simulink model "S1"  (R2014b)
settings: Solver=ode45  SolverMode=SingleTasking  StartTime=0.0  StopTime=100  MaxStep=5e-3  RelTol=1e-5  AbsTol=1e-5
values from neighbouring files (symbols this model uses):
  Domega = D_fw*Tb/w_b    (= 22.8676282526)    [m1.m]
  fixedFrequency = 0    [m1.m]
  genset = generators(1)    [m1.m]
  H = 5.6    [articlerun.m]    (also in m1.m = 0.5*J_rotor*wbasem*wbasem/Sbase)
  Ki = [-1/Xls 0       0       0       0       0       1/Xls   0 ... (first row only)    [articlerun.m]    (also in m1.m)
  Kmqmd = [ Xaq/Xls 0     0   Xaq/Xlkq2   0       0 ... (first row only)    [articlerun.m]    (also in m1.m = [ Xaq/Xls 0     0   Xaq/Xlkq2 0       0)
  Kpsi = [-rs/Xls 0     0       0       0       0       rs/Xls  0 ... (first row only)    [articlerun.m]    (also in m1.m = wb*Kpsi)
  Kv = [  1       0       0       0       0       0 ... (first row only)    [articlerun.m]    (also in m1.m = wb*Kv)
  Kwpsi = [0 -1   0   0   0   0 ... (first row only)    [articlerun.m]    (also in m1.m = zeros(6))
  psiInit = Psi.signals.values(end,1:7)    [articlerun.m]    (also in init.mat = [-391.464820784 14501.79303 -1.35791716672e-12 -350.14204148; m1.m = psiInit([1 2 3 5 6 7]))
  S_b = 325e6    (= 325000000)    [articlerun.m]    (also in m1.m)
  Sbase = S_b    (= 325000000)    [m1.m]
  ShortCircuitOn = 0    [articlerun.m]    (also in m1.m)
  ShortCircuitStart = 0    [articlerun.m]    (also in m1.m)
  ShortCircuitStop = 0    [articlerun.m]    (also in m1.m)
  swbId = 1    [initDrillingRigMSStoolboxMVM.m]
  Tb = S_b/w_b    (= 862089.275081)    [articlerun.m]    (also in m1.m)
  thetaInit = theta(end)*pi/180    [articlerun.m]    (also in init.mat = 0.0269876819053)
  V_b = 26e3    (= 26000)    [articlerun.m]    (also in m1.m = 20000)
  wb = 60*2*pi    (= 376.991118431)    [articlerun.m]    (also in m1.m)
undefined symbols (not defined in the file or in its folder): nr
undefined symbols (not defined in the file): generators
libraries: genset x4, powerlib x1
settings Model: Creator=andrdahl  LastModifiedBy=torsteinibo
settings DataIOCC: LimitDataPoints=off  SignalLoggingSaveFormat=ModelDataLogs  SaveOutput=off  DSMLogging=off  InspectSignalLogs=on  SaveTime=off
settings OptimizationCC: BlockReduction=off  BooleanDataType=off
settings DebuggingCC: SaveWithParameterizedLinksMsg=none  UnderspecifiedInitializationDetection=Classic  MergeDetectMultiDrivingBlocksExec=none  SignalResolutionControl=TryResolveAllWithWarning  SolverPrmCheckMsg=none  MultiTaskDSMMsg=warning  MultiTaskCondExecSysMsg=none  SignalLabelMismatchMsg=warning  StateNameClashWarn=warning  StrictBusMsg=WarnOnBusTreatedAsVector
settings HardwareCC: TargetUnknown=on
settings RTWCC: IncludeERTFirstTime=on

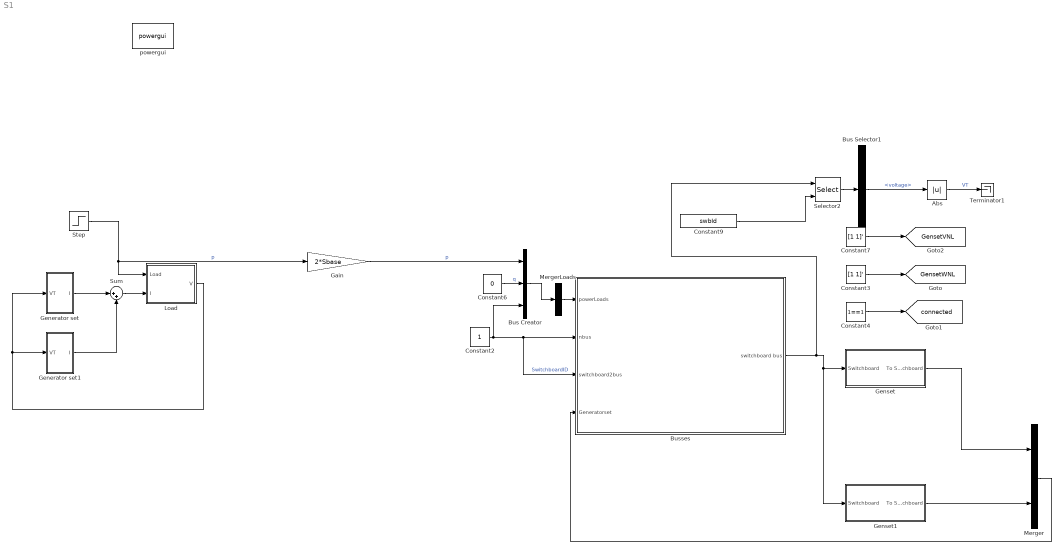
== system S1 ==
  Abs : Abs
  Bus Creator : BusCreator  Inputs='p','q','SwitchboardID'  OutDataTypeStr=Bus: powerLoadsBus  NonVirtualBus=on
  Bus Selector1 : BusSelector  OutputSignals=voltage
  Busses : Subsystem
      mask Display:
      | image(imread('figs/switchboard.jpg'))
      | port_label('input',1,'Power Loads')
      | port_label('input',2,'nbus')
      | port_label('input',3,'switchboard2bus')
      | port_label('input',4,'Generators')
      | port_label('output',1,'switchboard')
  Constant2 : Constant
  Constant3 : Constant  Value=[1 1]'
  Constant4 : Constant  Value=1==1
  Constant6 : Constant  Value=0
  Constant7 : Constant  Value=[1 1]'
  Constant9 : Constant  Value=swbId  OutDataTypeStr=Inherit: Inherit via back propagation
  Gain : Gain  Gain=2*Sbase
  Generator set : Subsystem
  Generator set1 : Subsystem
  Genset : Subsystem  mask{genset=generators(1)}
  Genset1 : Subsystem  mask{genset=generators(2)}
  Load : Subsystem
  Merger : Concatenate  Tag=FromGeneratorsetElectric/Merger
  MergerLoads : Concatenate  Tag=FromLoads/MergerLoads  NumInputs=1
  Selector2 : Selector  IndexOptions=Index vector (port)  Indices=[nr]
  Step : Step  Time=30  Before=.2  After=.7  SampleTime=0
  Sum : Sum  Inputs=|++
  Terminator1 : Terminator
  powergui : powerlib/powergui  Priority=1  SimulationMode=Continuous  SolverType=Tustin  SampleTime=50e-6  frequency=60  SPID=off  DisableSnubberDevices=off  DisableRonSwitches=off  DisableVfSwitches=off  SwTol=0  DisplayEquations=off  Interpol=off  methode=off  Ts=0  frequencyindice=60  Pbase=100e6  ErrMax=1e-4  Iterations=50  UnitsV=kV  UnitsW=MW  FunctionMessages=off  echomessages=off  HookPort=off  EnableUseOfTLC=off  x0status=blocks  RestoreLinks=warning  ResistiveCurrentMeasurement=off  Frange=[0:2:500]  Ylog=off  Xlog=on  ShowGrid=off  save=off  variable=ZData  structure=0  ZoomFFT=off  StartTime=0.0  cycles=1  DisplayStyle=1  fundamental=60  FreqAxis=off  MaxFrequency=1000  frequencyindicesteady=1  RmsSteady=1  display=off
  tag scope: GensetVNL=global, GensetWNL=global, connected=global
  wires:
  Merger/1 -> Busses/4(Generatorset)
  Genset1/1(To Switchboard) -> Merger/2
  Constant2/1 -> Bus Creator/3, Busses/3(switchboard2bus), Busses/2(nbus)  "SwitchboardID"
  Constant3/1 -> [GensetWNL]
  Constant4/1 -> [connected]
  MergerLoads/1 -> Busses/1(powerLoads)
  Bus Creator/1 -> MergerLoads/1
  Step/1 -> Gain/1, Load/1(Load)  "p"
  Constant6/1 -> Bus Creator/2  "q"
  Genset/1(To Switchboard) -> Merger/1
  Constant7/1 -> [GensetVNL]
  Constant9/1 -> Selector2/2
  Busses/1(switchboard bus) -> Selector2/1, Genset1/1(Switchboard), Genset/1(Switchboard)
  Selector2/1 -> Bus Selector1/1
  Bus Selector1/1 -> Abs/1  "<voltage>"
  Abs/1 -> Terminator1/1  "VT"
  Load/1(V) -> Generator set1/1(VT), Generator set/1(VT)
  Generator set/1(I) -> Sum/1
  Gain/1 -> Bus Creator/1  "p"
  Sum/1 -> Load/2(I)
  Generator set1/1(I) -> Sum/2

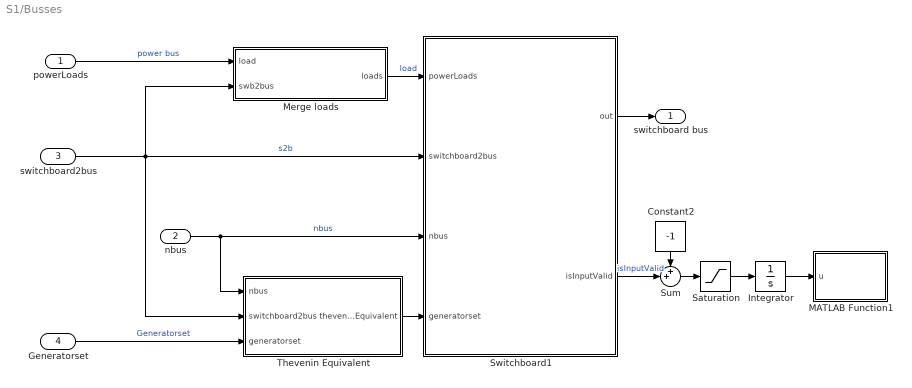
== system S1/Busses ==
  powerLoads : Inport  OutDataTypeStr=Bus: powerLoadsBus
  nbus : Inport  Port=2
  switchboard2bus : Inport  Port=3
  Generatorset : Inport  Port=4
  Constant2 : Constant  Value=-1
  Integrator : Integrator
  MATLAB Function1 : MATLAB Function  TreatAsAtomicUnit=on
  Merge loads : MATLAB Function  TreatAsAtomicUnit=on
  Saturation : Saturate  UpperLimit=0  LowerLimit=-1
  Sum : Sum  Inputs=++|
  Switchboard1 : MATLAB Function  TreatAsAtomicUnit=on
  Thevenin Equivalent : MATLAB Function  TreatAsAtomicUnit=on
  switchboard bus : Outport
  wires:
  Switchboard1/1(out) -> switchboard bus/1
  powerLoads/1 -> Merge loads/1(load)  "power bus"
  switchboard2bus/1 -> Thevenin Equivalent/2(switchboard2bus), Switchboard1/2(switchboard2bus), Merge loads/2(swb2bus)  "s2b"
  Generatorset/1 -> Thevenin Equivalent/3(generatorset)  "Generatorset"
  Integrator/1 -> MATLAB Function1/1(u)
  Constant2/1 -> Sum/1
  Sum/1 -> Saturation/1
  Switchboard1/2(isInputValid) -> Sum/2  "isInputValid"
  nbus/1 -> Thevenin Equivalent/1(nbus), Switchboard1/3(nbus)  "nbus"
  Merge loads/1(loads) -> Switchboard1/1(powerLoads)  "load"
  Thevenin Equivalent/1(theveninEquivalent) -> Switchboard1/4(generatorset)
  Saturation/1 -> Integrator/1

== system S1/Generator set ==
  VT : Inport
  AVR1 : Subsystem  AncestorBlock=PMSlib/Genset/AVR
  Demux4 : Demux  Outputs=3
  Embedded MATLAB Function : MATLAB Function  TreatAsAtomicUnit=on
  Embedded MATLAB Function1 : MATLAB Function  TreatAsAtomicUnit=on
  Embedded MATLAB Function2 : MATLAB Function  TreatAsAtomicUnit=on
  Generator : Subsystem
  Motor : Subsystem
  Product2 : Product  Multiplication=Matrix(*)  RndMeth=Zero
  Product3 : Product  Multiplication=Matrix(*)  RndMeth=Zero
  theta : Integrator  InitialCondition=thetaInit
  I : Outport
  wires:
  AVR1/1(Vf) -> Generator/3(Exfd)
  Product2/1 -> I/1
  Embedded MATLAB Function2/1(Vt) -> AVR1/2("V_T, Bus voltage")
  Embedded MATLAB Function1/1(Kinv) -> Product2/1
  Generator/3(Iqd0s) -> Product2/2
  theta/1 -> Embedded MATLAB Function1/1(theta), Embedded MATLAB Function/1(theta)
  Generator/4(Reactive power) -> AVR1/1("Q, reactive power")
  Generator/1(Electric torque) -> Motor/2(Electric torque)
  Motor/1(we) -> Generator/1(we), theta/1
  Embedded MATLAB Function/1(K) -> Product3/1
  Product3/1 -> Generator/2(Vqd0s)
  VT/1 -> Demux4/1, Product3/2
  Demux4/1 -> Embedded MATLAB Function2/1(Va)
  Demux4/2 -> Embedded MATLAB Function2/2(Vb)
  Demux4/3 -> Embedded MATLAB Function2/3(Vc)
  Generator/2(Active power) -> Motor/1(Active power)

== system S1/Generator set1 ==
  VT : Inport
  AVR1 : Subsystem  AncestorBlock=PMSlib/Genset/AVR
  Demux4 : Demux  Outputs=3
  Embedded MATLAB Function : MATLAB Function  TreatAsAtomicUnit=on
  Embedded MATLAB Function1 : MATLAB Function  TreatAsAtomicUnit=on
  Embedded MATLAB Function2 : MATLAB Function  TreatAsAtomicUnit=on
  Generator : Subsystem
  Motor : Subsystem
  Product2 : Product  Multiplication=Matrix(*)  RndMeth=Zero
  Product3 : Product  Multiplication=Matrix(*)  RndMeth=Zero
  theta : Integrator  InitialCondition=thetaInit
  I : Outport
  wires:
  AVR1/1(Vf) -> Generator/3(Exfd)
  Product2/1 -> I/1
  Embedded MATLAB Function2/1(Vt) -> AVR1/2("V_T, Bus voltage")
  Embedded MATLAB Function1/1(Kinv) -> Product2/1
  Generator/3(Iqd0s) -> Product2/2
  theta/1 -> Embedded MATLAB Function1/1(theta), Embedded MATLAB Function/1(theta)
  Generator/4(Reactive power) -> AVR1/1("Q, reactive power")
  Generator/1(Electric torque) -> Motor/2(Electric torque)
  Motor/1(we) -> Generator/1(we), theta/1
  Embedded MATLAB Function/1(K) -> Product3/1
  Product3/1 -> Generator/2(Vqd0s)
  VT/1 -> Demux4/1, Product3/2
  Demux4/1 -> Embedded MATLAB Function2/1(Va)
  Demux4/2 -> Embedded MATLAB Function2/2(Vb)
  Demux4/3 -> Embedded MATLAB Function2/3(Vc)
  Generator/2(Active power) -> Motor/1(Active power)

== system S1/Genset ==
  Switchboard : Inport
  Genset : Subsystem
  Terminator : Terminator
  To Switchboard : Outport
  wires:
  Genset/1(TheveninBus) -> To Switchboard/1
  Switchboard/1 -> Genset/1(Switchboard)
  Genset/2(GensetToPMS) -> Terminator/1

== system S1/Genset1 ==
  Switchboard : Inport
  Genset : Subsystem
  Terminator : Terminator
  To Switchboard : Outport
  wires:
  Genset/1(TheveninBus) -> To Switchboard/1
  Switchboard/1 -> Genset/1(Switchboard)
  Genset/2(GensetToPMS) -> Terminator/1

== system S1/Load ==
  Load : Inport
  I : Inport  Port=2
  Constant1 : Constant  Value=[0 0 0]
  Gain : Gain  Gain=2*S_b/V_b^2
  Product : Product  Inputs=*/  RndMeth=Zero
  Step1 : Step  Time=ShortCircuitStart  After=-ShortCircuitOn  SampleTime=0
  Step2 : Step  Time=ShortCircuitStop  After=ShortCircuitOn  SampleTime=0
  Sum1 : Sum  Inputs=|++
  Switch : Switch
  V : Outport
  wires:
  I/1 -> Product/1
  Load/1 -> Gain/1
  Product/1 -> Switch/1
  Sum1/1 -> Switch/2
  Step1/1 -> Sum1/1
  Step2/1 -> Sum1/2
  Constant1/1 -> Switch/3
  Switch/1 -> V/1
  Gain/1 -> Product/2

== system S1/Generator set/AVR1 ==
  "Q, reactive power" : Inport
  "V_T, Bus voltage" : Inport  Port=2
  AVR : Subsystem
  Gain1 : Gain  Gain=1/S_b
  Gain2 : Gain  Gain=1/V_b
  Gain3 : Gain  Gain=V_b*sqrt(2/3)
  Vf : Outport
  wires:
  "Q, reactive power"/1 -> Gain1/1
  "V_T, Bus voltage"/1 -> Gain2/1
  AVR/1(Vf) -> Gain3/1  "vf"
  Gain1/1 -> AVR/1("qe, pu")  "q"
  Gain2/1 -> AVR/2("V_T, pu")  "Vt"
  Gain3/1 -> Vf/1

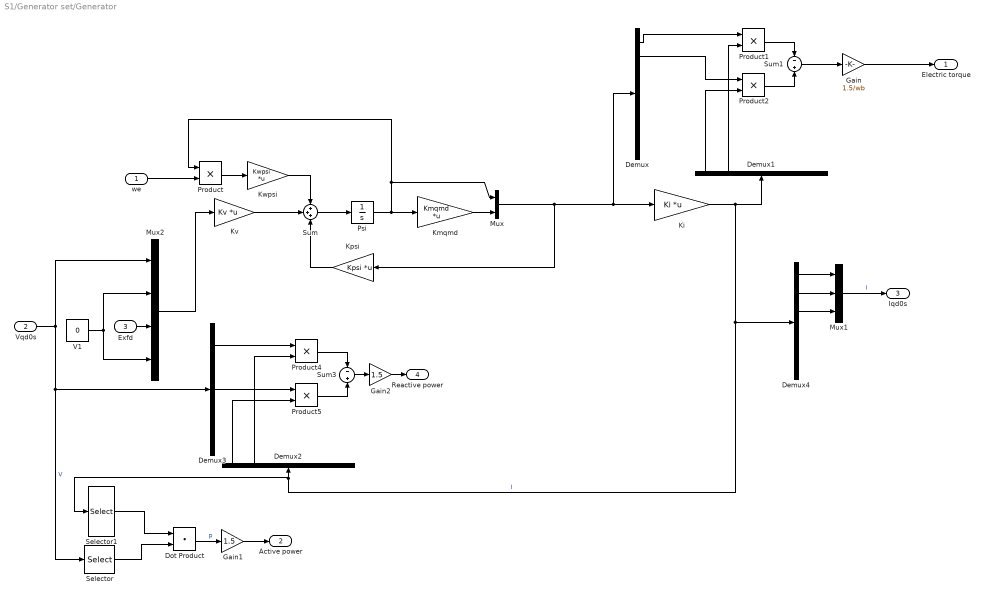
== system S1/Generator set/Generator ==
  we : Inport
  Vqd0s : Inport  Port=2
  Exfd : Inport  Port=3
  Demux : Demux  Outputs=8
  Demux1 : Demux  Outputs=6
  Demux2 : Demux  Outputs=6
  Demux3 : Demux  Outputs=3
  Demux4 : Demux  Outputs=6
  Dot Product : DotProduct  InputSameDT=on  OutDataTypeStr=Inherit: Inherit via internal rule
  Gain : Gain  Gain=1.5/wb
  Gain1 : Gain  Gain=1.5
  Gain2 : Gain  Gain=1.5
  Ki : Gain  Gain=Ki  Multiplication=Matrix(K*u)
  Kmqmd : Gain  Gain=Kmqmd  Multiplication=Matrix(K*u)
  Kpsi : Gain  Gain=Kpsi  Multiplication=Matrix(K*u)
  Kv : Gain  Gain=Kv  Multiplication=Matrix(K*u)
  Kwpsi : Gain  Gain=Kwpsi  Multiplication=Matrix(K*u)
  Mux : Mux  Inputs=2
  Mux1 : Mux  Inputs=3
  Mux2 : Mux
  Product{,1..2,4..5} (5 alike) : Product  RndMeth=Zero
  Psi : Integrator  InitialCondition=psiInit
  Selector : Selector  InputPortWidth=3  Indices=[1 2]
  Selector1 : Selector  InputPortWidth=6  Indices=[1 2]
  Sum : Sum  Inputs=+++
  Sum1 : Sum  Inputs=-+
  Sum3 : Sum  Inputs=-+
  V1 : Constant  Value=0
  Electric torque : Outport
  Active power : Outport  Port=2
  Iqd0s : Outport  Port=3
  Reactive power : Outport  Port=4
  wires:
  Psi/1 -> Kmqmd/1, Mux/1, Product/1
  Sum/1 -> Psi/1
  Product/1 -> Kwpsi/1
  Kwpsi/1 -> Sum/1
  Kv/1 -> Sum/2
  Kpsi/1 -> Sum/3
  Kmqmd/1 -> Mux/2
  Mux/1 -> Kpsi/1, Ki/1, Demux/1
  Ki/1 -> Demux1/1, Selector1/1, Demux2/1, Demux4/1  "I"
  Demux1/2 -> Product1/2
  Demux/1 -> Product1/1
  Demux/2 -> Product2/1
  Demux1/1 -> Product2/2
  Product2/1 -> Sum1/2
  Product1/1 -> Sum1/1
  Mux2/1 -> Kv/1
  Product5/1 -> Sum3/2
  Product4/1 -> Sum3/1
  Demux3/1 -> Product4/1
  Demux2/2 -> Product4/2
  V1/1 -> Mux2/4, Mux2/2
  we/1 -> Product/2
  Vqd0s/1 -> Selector/1, Demux3/1, Mux2/1  "V"
  Exfd/1 -> Mux2/3
  Sum1/1 -> Gain/1
  Sum3/1 -> Gain2/1
  Demux3/2 -> Product5/1
  Demux2/1 -> Product5/2
  Gain/1 -> Electric torque/1
  Demux4/1 -> Mux1/1
  Demux4/2 -> Mux1/2
  Demux4/3 -> Mux1/3
  Mux1/1 -> Iqd0s/1  "I"
  Selector/1 -> Dot Product/2
  Selector1/1 -> Dot Product/1
  Dot Product/1 -> Gain1/1  "p"
  Gain1/1 -> Active power/1
  Gain2/1 -> Reactive power/1

== system S1/Generator set/Motor ==
  Active power : Inport
  Electric torque : Inport  Port=2
  Governor1 : Subsystem
  Inertia : Gain  Gain=wb/(2*H*Tb)  Multiplication=Matrix(K*u)
  Inertia1 : Gain  Gain=1/S_b
  Inertia2 : Gain  Gain=Tb
  Inertia3 : Gain  Gain=1/wb
  Inertia4 : Gain  Gain=Domega  Multiplication=Matrix(K*u)
  Integrator1 : Integrator  InitialCondition=wb
  Sum2 : Sum  Inputs=--+
  we : Outport
  wires:
  Sum2/1 -> Inertia/1
  Inertia/1 -> Integrator1/1
  Integrator1/1 -> Inertia4/1, Inertia3/1, we/1
  Electric torque/1 -> Sum2/2
  Inertia3/1 -> Governor1/1(omega)  "w"
  Inertia2/1 -> Sum2/3
  Active power/1 -> Inertia1/1
  Inertia1/1 -> Governor1/2(P)  "p"
  Governor1/1(u) -> Inertia2/1
  Inertia4/1 -> Sum2/1

== system S1/Generator set1/AVR1 ==
  "Q, reactive power" : Inport
  "V_T, Bus voltage" : Inport  Port=2
  AVR : Subsystem
  Gain1 : Gain  Gain=1/S_b
  Gain2 : Gain  Gain=1/V_b
  Gain3 : Gain  Gain=V_b*sqrt(2/3)
  Vf : Outport
  wires:
  "Q, reactive power"/1 -> Gain1/1
  "V_T, Bus voltage"/1 -> Gain2/1
  AVR/1(Vf) -> Gain3/1  "vf"
  Gain1/1 -> AVR/1("qe, pu")  "q"
  Gain2/1 -> AVR/2("V_T, pu")  "Vt"
  Gain3/1 -> Vf/1

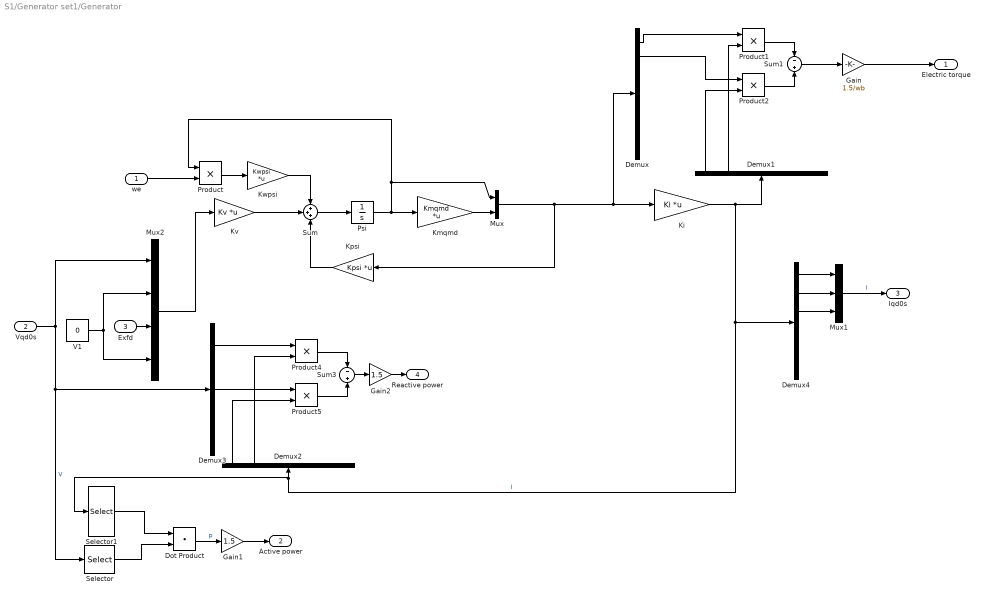
== system S1/Generator set1/Generator ==
  we : Inport
  Vqd0s : Inport  Port=2
  Exfd : Inport  Port=3
  Demux : Demux  Outputs=8
  Demux1 : Demux  Outputs=6
  Demux2 : Demux  Outputs=6
  Demux3 : Demux  Outputs=3
  Demux4 : Demux  Outputs=6
  Dot Product : DotProduct  InputSameDT=on  OutDataTypeStr=Inherit: Inherit via internal rule
  Gain : Gain  Gain=1.5/wb
  Gain1 : Gain  Gain=1.5
  Gain2 : Gain  Gain=1.5
  Ki : Gain  Gain=Ki  Multiplication=Matrix(K*u)
  Kmqmd : Gain  Gain=Kmqmd  Multiplication=Matrix(K*u)
  Kpsi : Gain  Gain=Kpsi  Multiplication=Matrix(K*u)
  Kv : Gain  Gain=Kv  Multiplication=Matrix(K*u)
  Kwpsi : Gain  Gain=Kwpsi  Multiplication=Matrix(K*u)
  Mux : Mux  Inputs=2
  Mux1 : Mux  Inputs=3
  Mux2 : Mux
  Product{,1..2,4..5} (5 alike) : Product  RndMeth=Zero
  Psi : Integrator  InitialCondition=psiInit
  Selector : Selector  InputPortWidth=3  Indices=[1 2]
  Selector1 : Selector  InputPortWidth=6  Indices=[1 2]
  Sum : Sum  Inputs=+++
  Sum1 : Sum  Inputs=-+
  Sum3 : Sum  Inputs=-+
  V1 : Constant  Value=0
  Electric torque : Outport
  Active power : Outport  Port=2
  Iqd0s : Outport  Port=3
  Reactive power : Outport  Port=4
  wires:
  Psi/1 -> Kmqmd/1, Mux/1, Product/1
  Sum/1 -> Psi/1
  Product/1 -> Kwpsi/1
  Kwpsi/1 -> Sum/1
  Kv/1 -> Sum/2
  Kpsi/1 -> Sum/3
  Kmqmd/1 -> Mux/2
  Mux/1 -> Kpsi/1, Ki/1, Demux/1
  Ki/1 -> Demux1/1, Selector1/1, Demux2/1, Demux4/1  "I"
  Demux1/2 -> Product1/2
  Demux/1 -> Product1/1
  Demux/2 -> Product2/1
  Demux1/1 -> Product2/2
  Product2/1 -> Sum1/2
  Product1/1 -> Sum1/1
  Mux2/1 -> Kv/1
  Product5/1 -> Sum3/2
  Product4/1 -> Sum3/1
  Demux3/1 -> Product4/1
  Demux2/2 -> Product4/2
  V1/1 -> Mux2/4, Mux2/2
  we/1 -> Product/2
  Vqd0s/1 -> Selector/1, Demux3/1, Mux2/1  "V"
  Exfd/1 -> Mux2/3
  Sum1/1 -> Gain/1
  Sum3/1 -> Gain2/1
  Demux3/2 -> Product5/1
  Demux2/1 -> Product5/2
  Gain/1 -> Electric torque/1
  Demux4/1 -> Mux1/1
  Demux4/2 -> Mux1/2
  Demux4/3 -> Mux1/3
  Mux1/1 -> Iqd0s/1  "I"
  Selector/1 -> Dot Product/2
  Selector1/1 -> Dot Product/1
  Dot Product/1 -> Gain1/1  "p"
  Gain1/1 -> Active power/1
  Gain2/1 -> Reactive power/1

== system S1/Generator set1/Motor ==
  Active power : Inport
  Electric torque : Inport  Port=2
  Governor1 : Subsystem
  Inertia : Gain  Gain=wb/(2*H*Tb)  Multiplication=Matrix(K*u)
  Inertia1 : Gain  Gain=1/S_b
  Inertia2 : Gain  Gain=Tb
  Inertia3 : Gain  Gain=1/wb
  Inertia4 : Gain  Gain=Domega  Multiplication=Matrix(K*u)
  Integrator1 : Integrator  InitialCondition=wb
  Sum2 : Sum  Inputs=--+
  we : Outport
  wires:
  Sum2/1 -> Inertia/1
  Inertia/1 -> Integrator1/1
  Integrator1/1 -> Inertia4/1, Inertia3/1, we/1
  Electric torque/1 -> Sum2/2
  Inertia3/1 -> Governor1/1(omega)  "w"
  Inertia2/1 -> Sum2/3
  Active power/1 -> Inertia1/1
  Inertia1/1 -> Governor1/2(P)  "p"
  Governor1/1(u) -> Inertia2/1
  Inertia4/1 -> Sum2/1

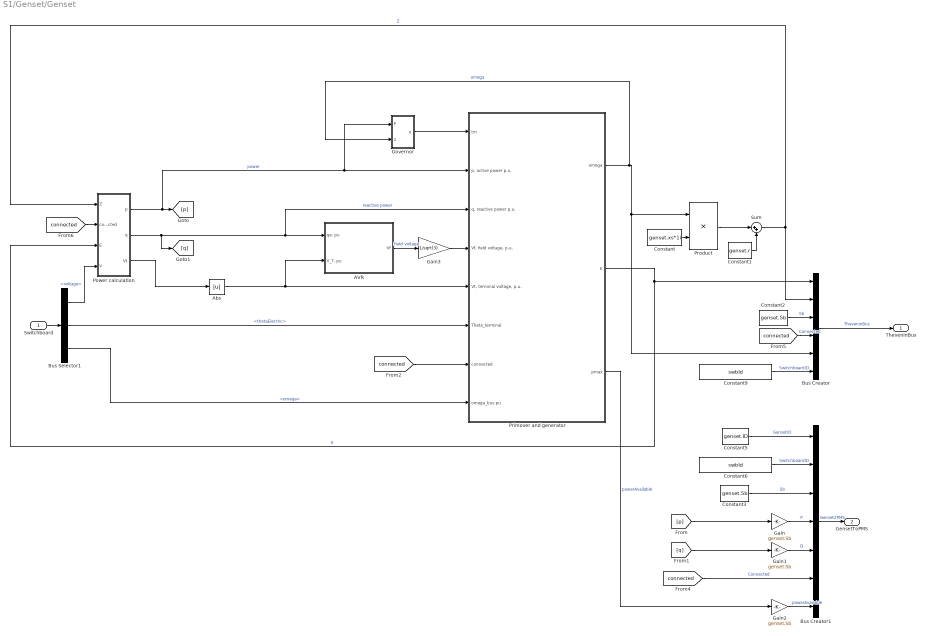
== system S1/Genset/Genset ==
  Switchboard : Inport
  AVR : Subsystem
  Abs : Abs
  Bus Creator : BusCreator  Inputs='E','Z','Sb','Connected','omega','SwitchboardID'  OutDataTypeStr=Bus: TheveninBus  NonVirtualBus=on
  Bus Creator1 : BusCreator  Inputs='GensetID','SwitchboardID','Sb','P','Q','Connected','powerAvailable'  OutDataTypeStr=Bus: Genset2PMS  NonVirtualBus=on
  Bus Selector1 : BusSelector  OutputSignals=voltage,thetaElectric,omega
  Constant : Constant  Value=genset.xs*1i
  Constant1 : Constant  Value=genset.r
  Constant2 : Constant  Value=genset.Sb
  Constant3 : Constant  Value=genset.Sb
  Constant5 : Constant  Value=genset.ID  OutDataTypeStr=Inherit: Inherit via back propagation
  Constant6 : Constant  Value=swbId  OutDataTypeStr=Inherit: Inherit via back propagation
  Constant9 : Constant  Value=swbId  OutDataTypeStr=Inherit: Inherit via back propagation
  Gain : Gain  Gain=genset.Sb
  Gain1 : Gain  Gain=genset.Sb
  Gain2 : Gain  Gain=genset.Sb
  Gain3 : Gain  Gain=1/sqrt(3)
  Governor : Subsystem
  Power calculation : MATLAB Function  TreatAsAtomicUnit=on
  Primover and generator : Subsystem
  Product : Product
  Sum : Sum  Inputs=|++
  TheveninBus : Outport
  GensetToPMS : Outport  Port=2
  wires:
  Bus Creator1/1 -> GensetToPMS/1  "Genset2PMS"
  [p] -> Gain/1
  [q] -> Gain1/1
  Constant2/1 -> Bus Creator/3  "Sb"
  Bus Creator/1 -> TheveninBus/1  "TheveninBus"
  Sum/1 -> Bus Creator/2, Power calculation/1(Z)  "Z"
  Constant1/1 -> Sum/2
  Product/1 -> Sum/1
  Constant/1 -> Product/2
  Abs/1 -> AVR/2("V_T, pu"), Primover and generator/5("Vt, terminal voltage, p.u.")
  Primover and generator/3(pmax) -> Gain2/1  "powerAvailable"
  Power calculation/2(q) -> [q], AVR/1("qe, pu"), Primover and generator/3("q, reactive power p.u.")  "reactive power"
  Power calculation/1(p) -> [p], Governor/1(P), Primover and generator/2("p, active power p.u.")  "power"
  Governor/1(u) -> Primover and generator/1(tm)
  Primover and generator/2(E) -> Power calculation/3(E), Bus Creator/1  "E"
  Primover and generator/1(omega) -> Governor/2(omega), Bus Creator/5, Product/1  "omega"
  AVR/1(Vf) -> Gain3/1  "Field voltage"
  Constant3/1 -> Bus Creator1/3  "Sb"
  Constant5/1 -> Bus Creator1/1  "GensetID"
  Constant6/1 -> Bus Creator1/2  "SwitchboardID"
  Gain/1 -> Bus Creator1/4  "P"
  Gain1/1 -> Bus Creator1/5  "Q"
  Bus Selector1/1 -> Power calculation/4(V)  "<voltage>"
  Gain2/1 -> Bus Creator1/7  "powerAvailable"
  [connected] -> Primover and generator/7(connected)
  [connected] -> Power calculation/2(connected)
  [connected] -> Bus Creator1/6  "Connected"
  [connected] -> Bus Creator/4  "Connected"
  Power calculation/3(Vt) -> Abs/1
  Bus Selector1/3 -> Primover and generator/8(omega_bus pu)  "<omega>"
  Switchboard/1 -> Bus Selector1/1
  Constant9/1 -> Bus Creator/6  "SwitchboardID"
  Bus Selector1/2 -> Primover and generator/6(Theta_terminal)  "<thetaElectric>"
  Gain3/1 -> Primover and generator/4("Vf, field voltage, p.u.")

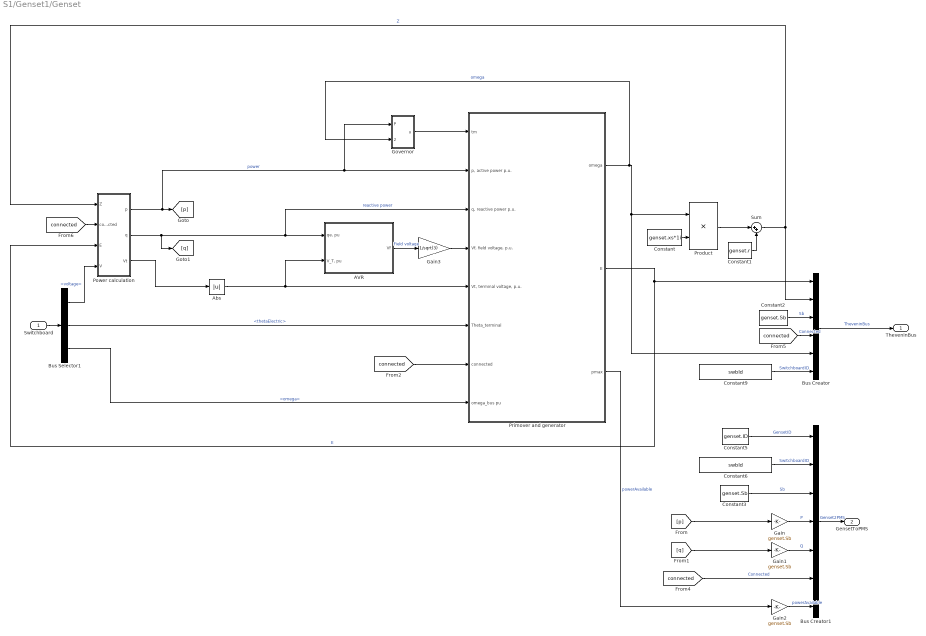
== system S1/Genset1/Genset ==
  Switchboard : Inport
  AVR : Subsystem
  Abs : Abs
  Bus Creator : BusCreator  Inputs='E','Z','Sb','Connected','omega','SwitchboardID'  OutDataTypeStr=Bus: TheveninBus  NonVirtualBus=on
  Bus Creator1 : BusCreator  Inputs='GensetID','SwitchboardID','Sb','P','Q','Connected','powerAvailable'  OutDataTypeStr=Bus: Genset2PMS  NonVirtualBus=on
  Bus Selector1 : BusSelector  OutputSignals=voltage,thetaElectric,omega
  Constant : Constant  Value=genset.xs*1i
  Constant1 : Constant  Value=genset.r
  Constant2 : Constant  Value=genset.Sb
  Constant3 : Constant  Value=genset.Sb
  Constant5 : Constant  Value=genset.ID  OutDataTypeStr=Inherit: Inherit via back propagation
  Constant6 : Constant  Value=swbId  OutDataTypeStr=Inherit: Inherit via back propagation
  Constant9 : Constant  Value=swbId  OutDataTypeStr=Inherit: Inherit via back propagation
  Gain : Gain  Gain=genset.Sb
  Gain1 : Gain  Gain=genset.Sb
  Gain2 : Gain  Gain=genset.Sb
  Gain3 : Gain  Gain=1/sqrt(3)
  Governor : Subsystem
  Power calculation : MATLAB Function  TreatAsAtomicUnit=on
  Primover and generator : Subsystem
  Product : Product
  Sum : Sum  Inputs=|++
  TheveninBus : Outport
  GensetToPMS : Outport  Port=2
  wires:
  Bus Creator1/1 -> GensetToPMS/1  "Genset2PMS"
  [p] -> Gain/1
  [q] -> Gain1/1
  Constant2/1 -> Bus Creator/3  "Sb"
  Bus Creator/1 -> TheveninBus/1  "TheveninBus"
  Sum/1 -> Bus Creator/2, Power calculation/1(Z)  "Z"
  Constant1/1 -> Sum/2
  Product/1 -> Sum/1
  Constant/1 -> Product/2
  Abs/1 -> AVR/2("V_T, pu"), Primover and generator/5("Vt, terminal voltage, p.u.")
  Primover and generator/3(pmax) -> Gain2/1  "powerAvailable"
  Power calculation/2(q) -> [q], AVR/1("qe, pu"), Primover and generator/3("q, reactive power p.u.")  "reactive power"
  Power calculation/1(p) -> [p], Governor/1(P), Primover and generator/2("p, active power p.u.")  "power"
  Governor/1(u) -> Primover and generator/1(tm)
  Primover and generator/2(E) -> Power calculation/3(E), Bus Creator/1  "E"
  Primover and generator/1(omega) -> Governor/2(omega), Bus Creator/5, Product/1  "omega"
  AVR/1(Vf) -> Gain3/1  "Field voltage"
  Constant3/1 -> Bus Creator1/3  "Sb"
  Constant5/1 -> Bus Creator1/1  "GensetID"
  Constant6/1 -> Bus Creator1/2  "SwitchboardID"
  Gain/1 -> Bus Creator1/4  "P"
  Gain1/1 -> Bus Creator1/5  "Q"
  Bus Selector1/1 -> Power calculation/4(V)  "<voltage>"
  Gain2/1 -> Bus Creator1/7  "powerAvailable"
  [connected] -> Primover and generator/7(connected)
  [connected] -> Power calculation/2(connected)
  [connected] -> Bus Creator1/6  "Connected"
  [connected] -> Bus Creator/4  "Connected"
  Power calculation/3(Vt) -> Abs/1
  Bus Selector1/3 -> Primover and generator/8(omega_bus pu)  "<omega>"
  Switchboard/1 -> Bus Selector1/1
  Constant9/1 -> Bus Creator/6  "SwitchboardID"
  Bus Selector1/2 -> Primover and generator/6(Theta_terminal)  "<thetaElectric>"
  Gain3/1 -> Primover and generator/4("Vf, field voltage, p.u.")

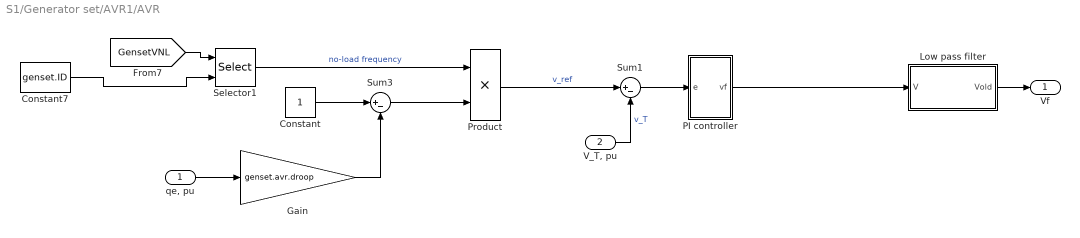
== system S1/Generator set/AVR1/AVR ==
  "qe, pu" : Inport
  "V_T, pu" : Inport  Port=2
  Constant : Constant
  Constant7 : Constant  Value=genset.ID  OutDataTypeStr=Inherit: Inherit via back propagation
  Gain : Gain  Gain=genset.avr.droop
  Low pass filter : Subsystem
  PI controller : Subsystem
  Product : Product  RndMeth=Zero
  Selector1 : Selector  IndexOptions=Index vector (port)  Indices=[nr]
  Sum1 : Sum  Inputs=|+-
  Sum3 : Sum  Inputs=|+-
  Vf : Outport
  wires:
  Low pass filter/1(Vold) -> Vf/1
  Product/1 -> Sum1/1  "v_ref"
  Sum3/1 -> Product/2
  Gain/1 -> Sum3/2
  Constant/1 -> Sum3/1
  "V_T, pu"/1 -> Sum1/2  "v_T"
  "qe, pu"/1 -> Gain/1
  Sum1/1 -> PI controller/1(e)
  Constant7/1 -> Selector1/2
  [GensetVNL] -> Selector1/1
  Selector1/1 -> Product/1  "no-load frequency"
  PI controller/1(vf) -> Low pass filter/1(V)

== system S1/Generator set/Motor/Governor1 ==
  omega : Inport
  P : Inport  Port=2
  Constant : Constant  Value=1/(1-genset.governor.droop*.5)
  Governor : genset/Genset/Governor
  u : Outport
  wires:
  P/1 -> Governor/4
  omega/1 -> Governor/2
  Constant/1 -> Governor/3
  Governor/1 -> u/1, Governor/1

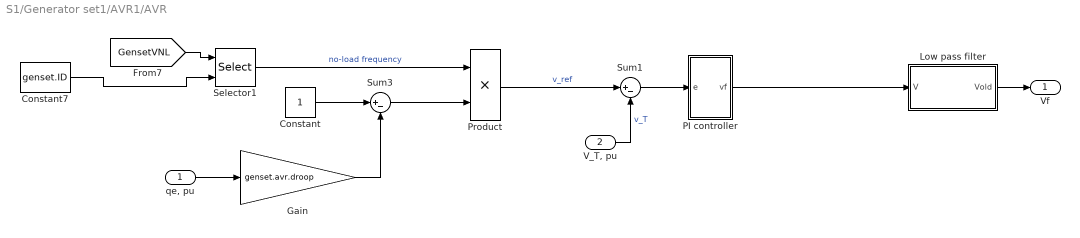
== system S1/Generator set1/AVR1/AVR ==
  "qe, pu" : Inport
  "V_T, pu" : Inport  Port=2
  Constant : Constant
  Constant7 : Constant  Value=genset.ID  OutDataTypeStr=Inherit: Inherit via back propagation
  Gain : Gain  Gain=genset.avr.droop
  Low pass filter : Subsystem
  PI controller : Subsystem
  Product : Product  RndMeth=Zero
  Selector1 : Selector  IndexOptions=Index vector (port)  Indices=[nr]
  Sum1 : Sum  Inputs=|+-
  Sum3 : Sum  Inputs=|+-
  Vf : Outport
  wires:
  Low pass filter/1(Vold) -> Vf/1
  Product/1 -> Sum1/1  "v_ref"
  Sum3/1 -> Product/2
  Gain/1 -> Sum3/2
  Constant/1 -> Sum3/1
  "V_T, pu"/1 -> Sum1/2  "v_T"
  "qe, pu"/1 -> Gain/1
  Sum1/1 -> PI controller/1(e)
  Constant7/1 -> Selector1/2
  [GensetVNL] -> Selector1/1
  Selector1/1 -> Product/1  "no-load frequency"
  PI controller/1(vf) -> Low pass filter/1(V)

== system S1/Generator set1/Motor/Governor1 ==
  omega : Inport
  P : Inport  Port=2
  Constant : Constant  Value=1/(1-genset.governor.droop*.5)
  Governor : genset/Genset/Governor
  u : Outport
  wires:
  P/1 -> Governor/4
  omega/1 -> Governor/2
  Constant/1 -> Governor/3
  Governor/1 -> u/1, Governor/1

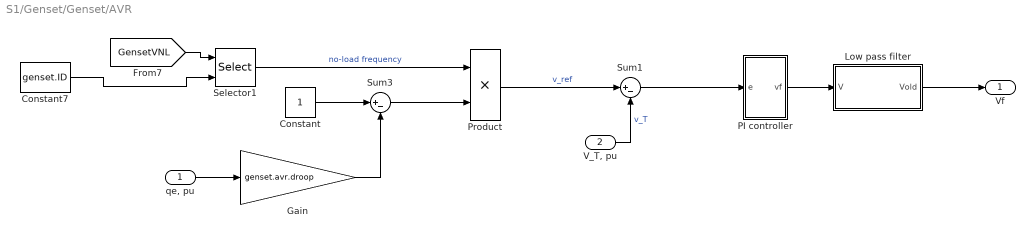
== system S1/Genset/Genset/AVR ==
  "qe, pu" : Inport
  "V_T, pu" : Inport  Port=2
  Constant : Constant
  Constant7 : Constant  Value=genset.ID  OutDataTypeStr=Inherit: Inherit via back propagation
  Gain : Gain  Gain=genset.avr.droop
  Low pass filter : Subsystem
  PI controller : Subsystem
  Product : Product  RndMeth=Zero
  Selector1 : Selector  IndexOptions=Index vector (port)  Indices=[nr]
  Sum1 : Sum  Inputs=|+-
  Sum3 : Sum  Inputs=|+-
  Vf : Outport
  wires:
  Low pass filter/1(Vold) -> Vf/1
  Product/1 -> Sum1/1  "v_ref"
  Sum3/1 -> Product/2
  Gain/1 -> Sum3/2
  Constant/1 -> Sum3/1
  "V_T, pu"/1 -> Sum1/2  "v_T"
  "qe, pu"/1 -> Gain/1
  Sum1/1 -> PI controller/1(e)
  PI controller/1(vf) -> Low pass filter/1(V)
  Constant7/1 -> Selector1/2
  [GensetVNL] -> Selector1/1
  Selector1/1 -> Product/1  "no-load frequency"

== system S1/Genset/Genset/Governor ==
  P : Inport
  omega : Inport  Port=2
  Constant : Constant  Value=1/(1-genset.governor.droop*.5)
  Governor : genset/Genset/Governor
  u : Outport
  wires:
  P/1 -> Governor/4
  omega/1 -> Governor/2
  Constant/1 -> Governor/3
  Governor/1 -> u/1, Governor/1

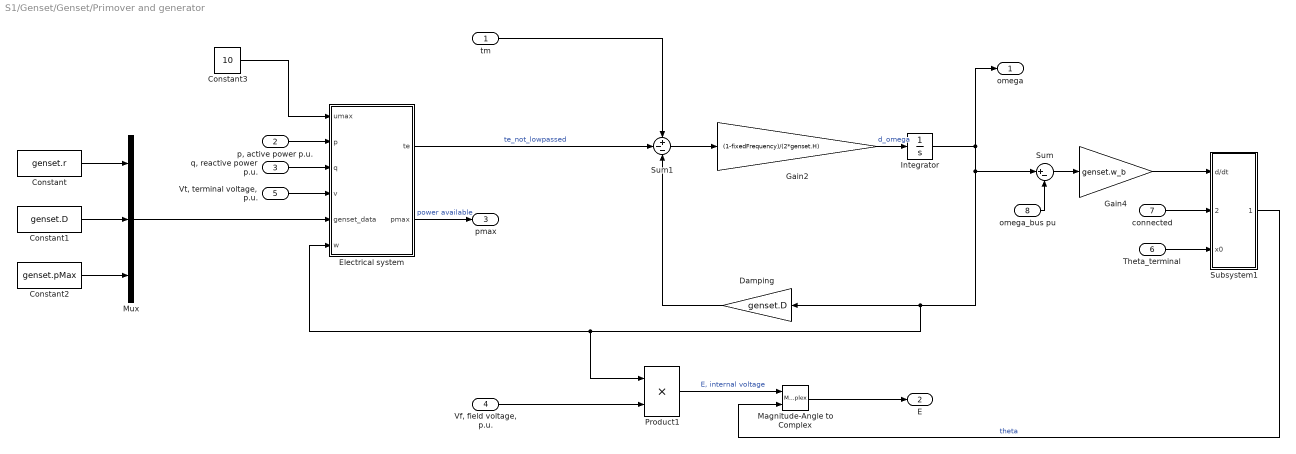
== system S1/Genset/Genset/Primover and generator ==
  tm : Inport
  "p, active power p.u." : Inport  Port=2
  "q, reactive power p.u." : Inport  Port=3
  "Vf, field voltage, p.u." : Inport  Port=4
  "Vt, terminal voltage, p.u." : Inport  Port=5
  Theta_terminal : Inport  Port=6
  connected : Inport  Port=7
  omega_bus pu : Inport  Port=8
  Constant : Constant  Value=genset.r
  Constant1 : Constant  Value=genset.D
  Constant2 : Constant  Value=genset.pMax
  Constant3 : Constant  Value=10
  Damping : Gain  Gain=genset.D
  Electrical system : MATLAB Function  TreatAsAtomicUnit=on
  Gain2 : Gain  Gain=(1-fixedFrequency)/(2*genset.H)
  Gain4 : Gain  Gain=genset.w_b
  Integrator : Integrator  InitialCondition=genset.omega0
  Magnitude-Angle to Complex : MagnitudeAngleToComplex
  Mux : Mux  Inputs=3
  Product1 : Product  Inputs=**  RndMeth=Zero
  Subsystem1 : Subsystem
  Sum : Sum  Inputs=|+-
  Sum1 : Sum  Inputs=+--
  omega : Outport
  E : Outport  Port=2
  pmax : Outport  Port=3
  wires:
  Mux/1 -> Electrical system/5(genset_data)
  Constant2/1 -> Mux/3
  Constant1/1 -> Mux/2
  Constant/1 -> Mux/1
  Magnitude-Angle to Complex/1 -> E/1
  Electrical system/2(pmax) -> pmax/1  "power available"
  Theta_terminal/1 -> Subsystem1/3(x0)
  Integrator/1 -> omega/1, Electrical system/6(w), Product1/1, Damping/1, Sum/1
  connected/1 -> Subsystem1/2(reset)
  Damping/1 -> Sum1/3
  "q, reactive power p.u."/1 -> Electrical system/3(q)
  "Vt, terminal voltage, p.u."/1 -> Electrical system/4(v)
  Electrical system/1(te) -> Sum1/2  "te_not_lowpassed"
  "p, active power p.u."/1 -> Electrical system/2(p)
  "Vf, field voltage, p.u."/1 -> Product1/2
  Gain2/1 -> Integrator/1  "d_omega"
  Sum1/1 -> Gain2/1
  Gain4/1 -> Subsystem1/1(d/dt)
  Subsystem1/1(Out1) -> Magnitude-Angle to Complex/2  "theta"
  Product1/1 -> Magnitude-Angle to Complex/1  "E, internal voltage"
  tm/1 -> Sum1/1
  Sum/1 -> Gain4/1
  omega_bus pu/1 -> Sum/2
  Constant3/1 -> Electrical system/1(umax)

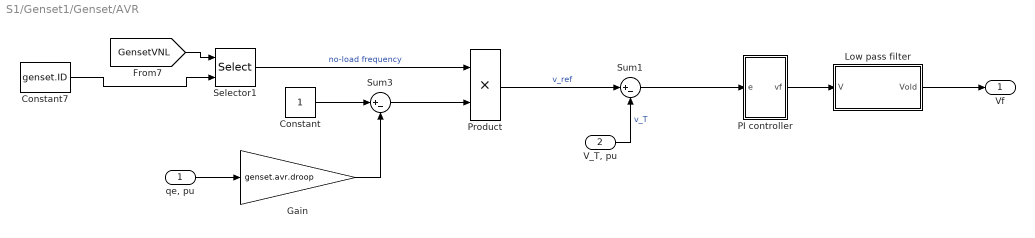
== system S1/Genset1/Genset/AVR ==
  "qe, pu" : Inport
  "V_T, pu" : Inport  Port=2
  Constant : Constant
  Constant7 : Constant  Value=genset.ID  OutDataTypeStr=Inherit: Inherit via back propagation
  Gain : Gain  Gain=genset.avr.droop
  Low pass filter : Subsystem
  PI controller : Subsystem
  Product : Product  RndMeth=Zero
  Selector1 : Selector  IndexOptions=Index vector (port)  Indices=[nr]
  Sum1 : Sum  Inputs=|+-
  Sum3 : Sum  Inputs=|+-
  Vf : Outport
  wires:
  Low pass filter/1(Vold) -> Vf/1
  Product/1 -> Sum1/1  "v_ref"
  Sum3/1 -> Product/2
  Gain/1 -> Sum3/2
  Constant/1 -> Sum3/1
  "V_T, pu"/1 -> Sum1/2  "v_T"
  "qe, pu"/1 -> Gain/1
  Sum1/1 -> PI controller/1(e)
  PI controller/1(vf) -> Low pass filter/1(V)
  Constant7/1 -> Selector1/2
  [GensetVNL] -> Selector1/1
  Selector1/1 -> Product/1  "no-load frequency"

== system S1/Genset1/Genset/Governor ==
  P : Inport
  omega : Inport  Port=2
  Constant : Constant  Value=1/(1-genset.governor.droop*.5)
  Governor : genset/Genset/Governor
  u : Outport
  wires:
  P/1 -> Governor/4
  omega/1 -> Governor/2
  Constant/1 -> Governor/3
  Governor/1 -> u/1, Governor/1

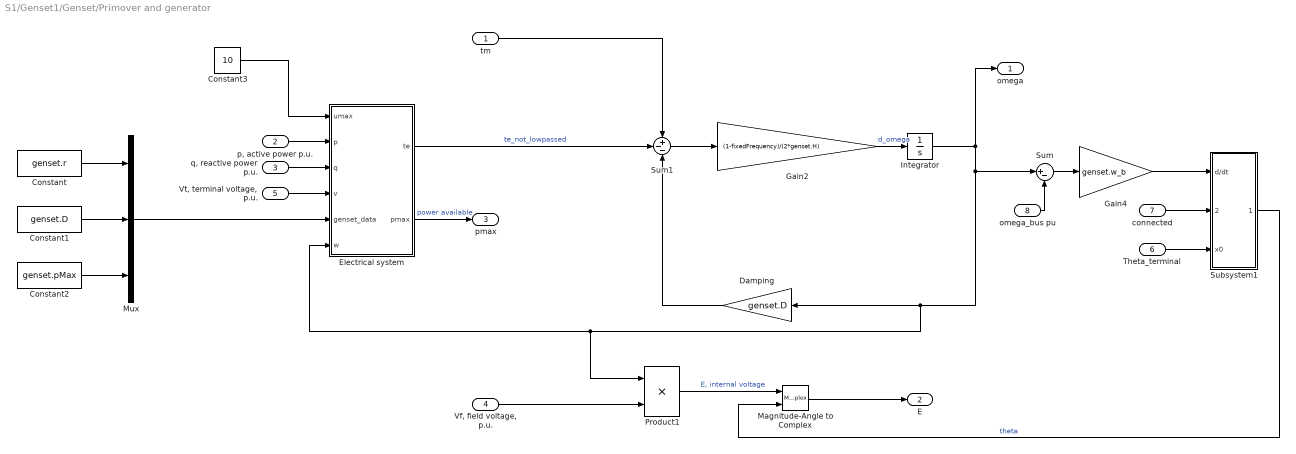
== system S1/Genset1/Genset/Primover and generator ==
  tm : Inport
  "p, active power p.u." : Inport  Port=2
  "q, reactive power p.u." : Inport  Port=3
  "Vf, field voltage, p.u." : Inport  Port=4
  "Vt, terminal voltage, p.u." : Inport  Port=5
  Theta_terminal : Inport  Port=6
  connected : Inport  Port=7
  omega_bus pu : Inport  Port=8
  Constant : Constant  Value=genset.r
  Constant1 : Constant  Value=genset.D
  Constant2 : Constant  Value=genset.pMax
  Constant3 : Constant  Value=10
  Damping : Gain  Gain=genset.D
  Electrical system : MATLAB Function  TreatAsAtomicUnit=on
  Gain2 : Gain  Gain=(1-fixedFrequency)/(2*genset.H)
  Gain4 : Gain  Gain=genset.w_b
  Integrator : Integrator  InitialCondition=genset.omega0
  Magnitude-Angle to Complex : MagnitudeAngleToComplex
  Mux : Mux  Inputs=3
  Product1 : Product  Inputs=**  RndMeth=Zero
  Subsystem1 : Subsystem
  Sum : Sum  Inputs=|+-
  Sum1 : Sum  Inputs=+--
  omega : Outport
  E : Outport  Port=2
  pmax : Outport  Port=3
  wires:
  Mux/1 -> Electrical system/5(genset_data)
  Constant2/1 -> Mux/3
  Constant1/1 -> Mux/2
  Constant/1 -> Mux/1
  Magnitude-Angle to Complex/1 -> E/1
  Electrical system/2(pmax) -> pmax/1  "power available"
  Theta_terminal/1 -> Subsystem1/3(x0)
  Integrator/1 -> omega/1, Electrical system/6(w), Product1/1, Damping/1, Sum/1
  connected/1 -> Subsystem1/2(reset)
  Damping/1 -> Sum1/3
  "q, reactive power p.u."/1 -> Electrical system/3(q)
  "Vt, terminal voltage, p.u."/1 -> Electrical system/4(v)
  Electrical system/1(te) -> Sum1/2  "te_not_lowpassed"
  "p, active power p.u."/1 -> Electrical system/2(p)
  "Vf, field voltage, p.u."/1 -> Product1/2
  Gain2/1 -> Integrator/1  "d_omega"
  Sum1/1 -> Gain2/1
  Gain4/1 -> Subsystem1/1(d/dt)
  Subsystem1/1(Out1) -> Magnitude-Angle to Complex/2  "theta"
  Product1/1 -> Magnitude-Angle to Complex/1  "E, internal voltage"
  tm/1 -> Sum1/1
  Sum/1 -> Gain4/1
  omega_bus pu/1 -> Sum/2
  Constant3/1 -> Electrical system/1(umax)

== system S1/Generator set/AVR1/AVR/Low pass filter ==
  V : Inport
  Gain : Gain  Gain=1/genset.avr.T
  Integrator : Integrator  InitialCondition=genset.avr.v0
  Sum : Sum  Inputs=|+-
  Vold : Outport
  wires:
  Gain/1 -> Integrator/1
  Sum/1 -> Gain/1
  V/1 -> Sum/1
  Integrator/1 -> Sum/2, Vold/1

== system S1/Generator set/AVR1/AVR/PI controller ==
  e : Inport
  Gain1 : Gain  Gain=genset.avr.kp
  Gain2 : Gain  Gain=genset.avr.ki
  Integrator : Integrator
  Saturation : Saturate  UpperLimit=genset.avr.maxFieldVoltage  LowerLimit=genset.avr.minFieldVoltage  LinearizeAsGain=off  OutMin=genset.avr.minFieldVoltage  OutMax=genset.avr.maxFieldVoltage  OutDataTypeStr=Inherit: Inherit via back propagation
  Sum : Sum  Inputs=|++
  vf : Outport
  wires:
  e/1 -> Gain2/1, Gain1/1
  Saturation/1 -> vf/1
  Gain1/1 -> Sum/1
  Gain2/1 -> Integrator/1
  Integrator/1 -> Sum/2
  Sum/1 -> Saturation/1

== system S1/Generator set1/AVR1/AVR/Low pass filter ==
  V : Inport
  Gain : Gain  Gain=1/genset.avr.T
  Integrator : Integrator  InitialCondition=genset.avr.v0
  Sum : Sum  Inputs=|+-
  Vold : Outport
  wires:
  Gain/1 -> Integrator/1
  Sum/1 -> Gain/1
  V/1 -> Sum/1
  Integrator/1 -> Sum/2, Vold/1

== system S1/Generator set1/AVR1/AVR/PI controller ==
  e : Inport
  Gain1 : Gain  Gain=genset.avr.kp
  Gain2 : Gain  Gain=genset.avr.ki
  Integrator : Integrator
  Saturation : Saturate  UpperLimit=genset.avr.maxFieldVoltage  LowerLimit=genset.avr.minFieldVoltage  LinearizeAsGain=off  OutMin=genset.avr.minFieldVoltage  OutMax=genset.avr.maxFieldVoltage  OutDataTypeStr=Inherit: Inherit via back propagation
  Sum : Sum  Inputs=|++
  vf : Outport
  wires:
  e/1 -> Gain2/1, Gain1/1
  Saturation/1 -> vf/1
  Gain1/1 -> Sum/1
  Gain2/1 -> Integrator/1
  Integrator/1 -> Sum/2
  Sum/1 -> Saturation/1

== system S1/Genset/Genset/AVR/Low pass filter ==
  V : Inport
  Gain : Gain  Gain=1/genset.avr.T
  Integrator : Integrator  InitialCondition=genset.avr.v0
  Sum : Sum  Inputs=|+-
  Vold : Outport
  wires:
  Gain/1 -> Integrator/1
  Sum/1 -> Gain/1
  V/1 -> Sum/1
  Integrator/1 -> Sum/2, Vold/1

== system S1/Genset/Genset/AVR/PI controller ==
  e : Inport
  Gain2 : Gain  Gain=genset.avr.kp
  Gain3 : Gain  Gain=genset.avr.ki
  Integrator : Integrator
  Saturation : Saturate  UpperLimit=genset.avr.maxFieldVoltage  LowerLimit=genset.avr.minFieldVoltage  LinearizeAsGain=off  OutMin=genset.avr.minFieldVoltage  OutMax=genset.avr.maxFieldVoltage  OutDataTypeStr=Inherit: Inherit via back propagation
  Sum : Sum  Inputs=|++
  vf : Outport
  wires:
  Saturation/1 -> vf/1
  e/1 -> Gain3/1, Gain2/1
  Gain2/1 -> Sum/1
  Gain3/1 -> Integrator/1
  Integrator/1 -> Sum/2
  Sum/1 -> Saturation/1

== system S1/Genset/Genset/Primover and generator/Subsystem1 ==
  d/dt : Inport
  reset : Inport  Port=2
  x0 : Inport  Port=3
  Gain : Gain  Gain=1000
  Integrator : Integrator  InitialCondition=genset.theta0
  MATLAB Function : MATLAB Function  TreatAsAtomicUnit=on
  Sum : Sum  Inputs=-|+
  Switch : Switch  Threshold=1
  Out1 : Outport
  wires:
  Switch/1 -> Integrator/1
  d/dt/1 -> Switch/1
  MATLAB Function/1(y) -> Gain/1
  Gain/1 -> Switch/3
  Sum/1 -> MATLAB Function/1(u)
  x0/1 -> Sum/2
  reset/1 -> Switch/2
  Integrator/1 -> Sum/1, Out1/1

== system S1/Genset1/Genset/AVR/Low pass filter ==
  V : Inport
  Gain : Gain  Gain=1/genset.avr.T
  Integrator : Integrator  InitialCondition=genset.avr.v0
  Sum : Sum  Inputs=|+-
  Vold : Outport
  wires:
  Gain/1 -> Integrator/1
  Sum/1 -> Gain/1
  V/1 -> Sum/1
  Integrator/1 -> Sum/2, Vold/1

== system S1/Genset1/Genset/AVR/PI controller ==
  e : Inport
  Gain1 : Gain  Gain=genset.avr.kp
  Gain2 : Gain  Gain=genset.avr.ki
  Integrator : Integrator
  Saturation : Saturate  UpperLimit=genset.avr.maxFieldVoltage  LowerLimit=genset.avr.minFieldVoltage  LinearizeAsGain=off  OutMin=genset.avr.minFieldVoltage  OutMax=genset.avr.maxFieldVoltage  OutDataTypeStr=Inherit: Inherit via back propagation
  Sum : Sum  Inputs=|++
  vf : Outport
  wires:
  Saturation/1 -> vf/1
  e/1 -> Gain2/1, Gain1/1
  Gain1/1 -> Sum/1
  Gain2/1 -> Integrator/1
  Integrator/1 -> Sum/2
  Sum/1 -> Saturation/1

== system S1/Genset1/Genset/Primover and generator/Subsystem1 ==
  d/dt : Inport
  reset : Inport  Port=2
  x0 : Inport  Port=3
  Gain : Gain  Gain=1000
  Integrator : Integrator  InitialCondition=genset.theta0
  MATLAB Function : MATLAB Function  TreatAsAtomicUnit=on
  Sum : Sum  Inputs=-|+
  Switch : Switch  Threshold=1
  Out1 : Outport
  wires:
  Switch/1 -> Integrator/1
  d/dt/1 -> Switch/1
  MATLAB Function/1(y) -> Gain/1
  Gain/1 -> Switch/3
  Sum/1 -> MATLAB Function/1(u)
  x0/1 -> Sum/2
  reset/1 -> Switch/2
  Integrator/1 -> Sum/1, Out1/1

== matlab function S1/Busses/MATLAB Function1 ==
  data: u input
function stopper(u)
%#codegen
if ( u < -1)
    error('Bus voltage calculations have been invalid for 1 second, stopping stimulation');
end

== matlab function S1/Genset/Genset/Primover and generator/Electrical system ==
  data: umax input; p input size=1; q input; v input; genset_data input; te output; w input; pmax output size=1
function [te,pmax] = fcn(umax,p,q,v,genset_data,w)
r     = genset_data(1);
D     = genset_data(2);
p_max = genset_data(3);

te = (p+r*(p^2+q^2)/v^2)/w;
pmax = min((v/(1+r))*(-D*w^2+umax*w-r*q^2/v),p_max);

== matlab function S1/Busses/Merge loads ==
  data: load input; loads output Bus: powerLoadsBus; swb2bus input
function loads  = mergeloads(load,swb2bus)
%#codegen
loads = repmat( struct( 'p',0,'q',0,'SwitchboardID',0),length(swb2bus),1);
for i = 1:length(load)
    bus = swb2bus(load(i).SwitchboardID);
    loads(bus).p = loads(bus).p+ load(i).p;
    loads(bus).q = loads(bus).q+ load(i).q;
end
for i = 1:length(swb2bus)
    loads(i).SwitchboardID = i;
end

== matlab function S1/Genset1/Genset/Power calculation ==
  data: Z input; connected input; p output; E input; V input; q output; Vt output
function [p,q,Vt] = power(Z,connected,E,V)
%#codegen
if (connected)
Vt = V;
V = V/sqrt(3);
s = 3*V.*conj((E-V)./Z);
p = real(s);
q = imag(s);

else
p = 0;
q = 0;
Vt =E*sqrt(3);
end

== matlab function S1/Genset1/Genset/Primover and generator/Electrical system ==
  data: umax input; p input size=1; q input; v input; genset_data input; te output; w input; pmax output size=1
function [te,pmax] = fcn(umax,p,q,v,genset_data,w)
r     = genset_data(1);
D     = genset_data(2);
p_max = genset_data(3);

te = (p+r*(p^2+q^2)/v^2)/w;
pmax = min((v/(1+r))*(-D*w^2+umax*w-r*q^2/v),p_max);

== matlab function S1/Busses/Switchboard1 ==
  data: powerLoads input; out output Bus: swb; isInputValid output size=1; switchboard2bus input; nbus input; generatorset input
function [out, isInputValid]= switchboard(powerLoads,switchboard2bus,nbus,generatorset)
%#codegen

[out, isInputValid]= switchboardCentral(powerLoads,switchboard2bus,nbus,generatorset);

== matlab function S1/Genset/Genset/Power calculation ==
  data: Z input; connected input; p output; E input; V input; q output; Vt output
function [p,q,Vt] = power(Z,connected,E,V)
%#codegen
if (connected)
Vt = V;
V = V/sqrt(3);
s = 3*V.*conj((E-V)./Z);
p = real(s);
q = imag(s);

else
p = 0;
q = 0;
Vt =E*sqrt(3);
end

== matlab function S1/Busses/Thevenin Equivalent ==
  data: nbus input; switchboard2bus input; generatorset input; theveninEquivalent output Bus: TheveninBus
function theveninEquivalent  = mergeGenerators(nbus,switchboard2bus,generatorset)
%#codegen
nSwitchboards = length(switchboard2bus);
assert(nbus<=nSwitchboards);
nGeneratorset = length(generatorset);
E = complex(zeros(nGeneratorset,1));
Z = complex(zeros(nGeneratorset,1));
Sb = zeros(nGeneratorset,1);
Connected = zeros(nGeneratorset,1);
omega = zeros(nGeneratorset,1);
genset2swb = zeros(nGeneratorset,1);
for i = 1:nGeneratorset
    E(i) = generatorset(i).E;
    Z(i) = generatorset(i).Z;
    Sb(i) = generatorset(i).Sb;
    Connected(i) = generatorset(i).Connected;
    omega(i) = generatorset(i).omega;
    genset2swb(i) = generatorset(i).SwitchboardID;
end   

theveninEquivalent = repmat( struct( 'E',1j,'Z',1j,'Sb',0,'Connected',true,'omega',0,'SwitchboardID',0),nSwitchboards);
for bus = 1:nbus
    %Find gensets connected to bus
    m = 0;  
    for i = 1:nGeneratorset
        if (switchboard2bus(genset2swb(i))==bus && Connected(i))
            m = m + 1;
        end
    end
    assert(m <= nGeneratorset);
    gensets = zeros(1,m);
    m = 0;    
    for i = 1:nGeneratorset
        if (switchboard2bus(genset2swb(i))==bus && Connected(i))
            m = m + 1;
            gensets(m) = i;
        end
    end
    [ et, zt, Sb_bus, ~, omegaAvgBus ] = TheveninEquivalent( E(gensets), Z(gensets), Sb(gensets), Connected(gensets), omega(gensets) );
    theveninEquivalent(bus).E = et;
    theveninEquivalent(bus).Z = zt;
    theveninEquivalent(bus).Sb = Sb_bus;
    theveninEquivalent(bus).Connected = true;
    theveninEquivalent(bus).omega = omegaAvgBus;
    theveninEquivalent(bus).SwitchboardID = bus;
end

== matlab function S1/Genset1/Genset/Primover and generator/Subsystem1/MATLAB Function ==
  data: u input; y output
function y = fcn(u)
%#codegen

y = anglemap(u);

== matlab function S1/Generator set/Embedded MATLAB Function ==
  data: theta input; K output
function K = Rotation(theta)

K = 2/3*[cos(theta) cos(theta-2*pi/3) cos(theta+2*pi/3)
         sin(theta) sin(theta-2*pi/3) sin(theta+2*pi/3)
         .5         .5                 .5];

== matlab function S1/Generator set/Embedded MATLAB Function1 ==
  data: theta input; Kinv output
function Kinv = RotationInv(theta)

Kinv = [cos(theta)         sin(theta)      1
     cos(theta-2*pi/3)  sin(theta-2*pi/3)   1
     cos(theta+2*pi/3)  sin(theta+2*pi/3)   1];

== matlab function S1/Generator set/Embedded MATLAB Function2 ==
  data: Va input; Vt output; Vb input; Vc input; theta output
function [Vt,theta] = LengthV(Va, Vb, Vc)

Vb = Vb*exp(2/3*pi*1j);
Vc = Vc*exp(-2/3*pi*1j);

V = Va+Vb+Vc;

Vt = abs(V)*sqrt(2/3);
theta = angle(V);

== matlab function S1/Generator set1/Embedded MATLAB Function ==
  data: theta input; K output
function K = Rotation(theta)

K = 2/3*[cos(theta) cos(theta-2*pi/3) cos(theta+2*pi/3)
         sin(theta) sin(theta-2*pi/3) sin(theta+2*pi/3)
         .5         .5                 .5];

== matlab function S1/Generator set1/Embedded MATLAB Function1 ==
  data: theta input; Kinv output
function Kinv = RotationInv(theta)

Kinv = [cos(theta)         sin(theta)      1
     cos(theta-2*pi/3)  sin(theta-2*pi/3)   1
     cos(theta+2*pi/3)  sin(theta+2*pi/3)   1];

== matlab function S1/Generator set1/Embedded MATLAB Function2 ==
  data: Va input; Vt output; Vb input; Vc input; theta output
function [Vt,theta] = LengthV(Va, Vb, Vc)

Vb = Vb*exp(2/3*pi*1j);
Vc = Vc*exp(-2/3*pi*1j);

V = Va+Vb+Vc;

Vt = abs(V)*sqrt(2/3);
theta = angle(V);

== matlab function S1/Genset/Genset/Primover and generator/Subsystem1/MATLAB Function ==
  data: u input; y output
function y = fcn(u)
%#codegen

y = anglemap(u);
